simulink model "Ex2s"  (R2025a)
settings: Solver=VariableStepAuto  StartTime=0.0  StopTime=10.0  RelTol=1e-3
values from neighbouring files (symbols this model uses):
  A = [0 1 ; -25 -4]    [Ex2.m]
  B = [1 1 ; 0 1]    [Ex2.m]
  C = [1 0 ; 0 1]    [Ex2.m]
  D = [0 0 ; 0 0]    [Ex2.m]
  Gp = [g11 g12;g21 g22]    [Ex1.m]    (also in Ex2.m = tf(sys))

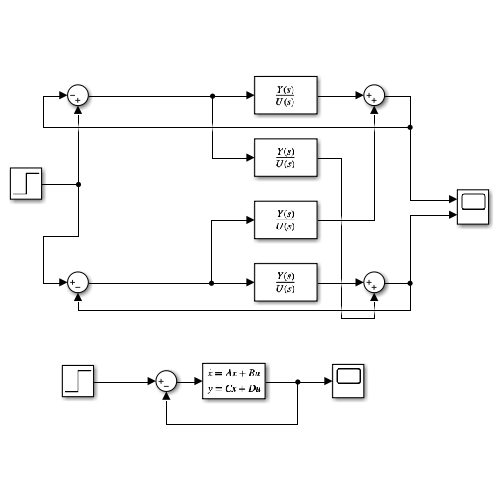
[thumbnail: Simulink's stored preview of the top-level diagram]
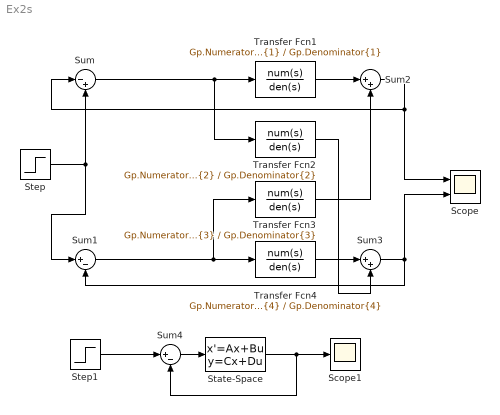
== system Ex2s ==
  Scope : Scope  NumInputPorts=2
      settings: ActiveDisplayYMinimum=-11.298922582324753  ActiveDisplayYMaximum=4.9604863402073729
  Scope1 : Scope
      settings: ActiveDisplayYMinimum=-10.034819620525726  ActiveDisplayYMaximum=5.3274041998970629
  State-Space : StateSpace  A=A  B=B  C=C  D=D  InitialCondition=0
  Step : Step  SampleTime=0
  Step1 : Step  SampleTime=0
  Sum : Sum  Inputs=|-+
  Sum1 : Sum  Inputs=|+-
  Sum2 : Sum  Inputs=|++
  Sum3 : Sum  Inputs=|++
  Sum4 : Sum  Inputs=|+-
  Transfer Fcn1 : TransferFcn  Numerator=Gp.Numerator{1}  Denominator=Gp.Denominator{1}
  Transfer Fcn2 : TransferFcn  Numerator=Gp.Numerator{2}  Denominator=Gp.Denominator{2}
  Transfer Fcn3 : TransferFcn  Numerator=Gp.Numerator{3}  Denominator=Gp.Denominator{3}
  Transfer Fcn4 : TransferFcn  Numerator=Gp.Numerator{4}  Denominator=Gp.Denominator{4}
  wires:
  Sum3/1 -> Scope/2, Sum1/2
  Sum2/1 -> Scope/1, Sum/1
  Sum/1 -> Transfer Fcn2/1, Transfer Fcn1/1
  Step/1 -> Sum/2, Sum1/1
  Sum1/1 -> Transfer Fcn4/1, Transfer Fcn3/1
  Transfer Fcn1/1 -> Sum2/1
  Transfer Fcn2/1 -> Sum3/2
  Transfer Fcn3/1 -> Sum2/2
  Transfer Fcn4/1 -> Sum3/1
  Step1/1 -> Sum4/1
  Sum4/1 -> State-Space/1
  State-Space/1 -> Sum4/2, Scope1/1
